simulink model "test_sim"  (R2022b)
settings: Solver=ode4  StartTime=0.0  StopTime=10  FixedStep=0.001  RelTol=1e-3
settings Model: Creator=user  LastModifiedBy=user
settings DataIOCC: ReturnWorkspaceOutputs=off

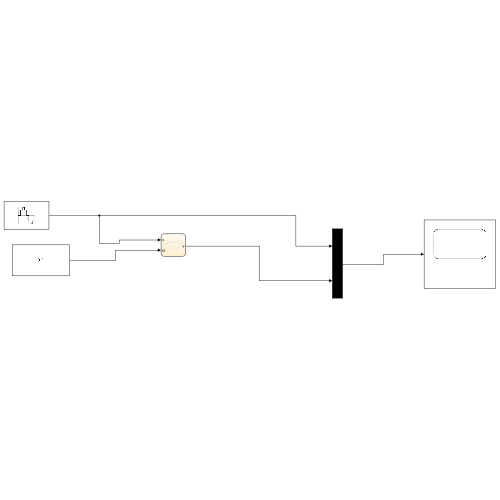
[thumbnail: Simulink's stored preview of the top-level diagram]
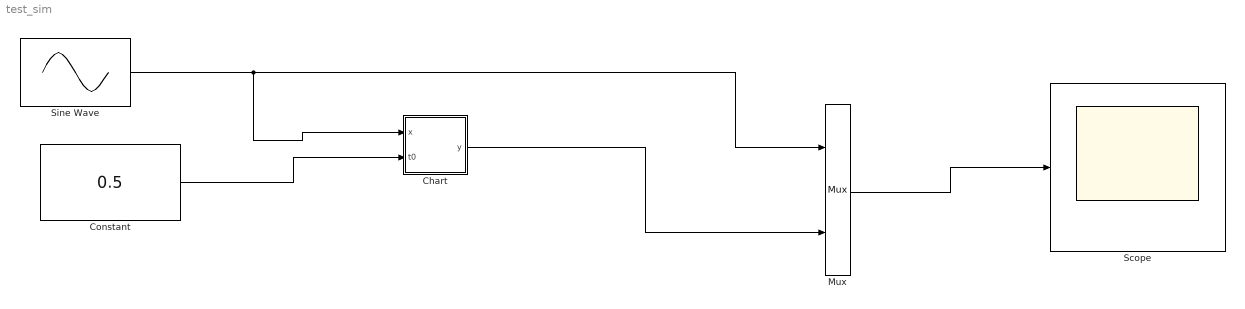
== system test_sim ==
  Chart : Stateflow chart  TreatAsAtomicUnit=on
  Constant : Constant  Value=0.5
  Mux : Mux  Inputs=2
  Scope : Scope
  Sine Wave : Sin  SampleTime=0.01
  wires:
  Constant/1 -> Chart/2(t0)
  Sine Wave/1 -> Chart/1(x), Mux/1
  Chart/1(y) -> Mux/2
  Mux/1 -> Scope/1

== stateflow chart test_sim/Chart ==
  state Mode1
    y=1;
  state Mode2
    y=-1;
  state Mode3
    y=0;
  Mode1 -> Mode2 [order 1] : [x<-t0]
  Mode2 -> Mode1 [order 1] : [x>=t0]
  Mode3 -> Mode1 [order 1] : [x>=t0]
  Mode1 -> Mode3 [order 2] : [abs(x) < t0]
  Mode3 -> Mode2 [order 2] : [x<=-t0]
  Mode2 -> Mode3 [order 2] : [abs(x)<t0]
  (default) -> Mode3
  data: y output; x input; t0 input
